simulink model "Week2_Problem3"  (R2020a)
settings: Solver=VariableStepAuto  StartTime=0.0  StopTime=10.0  RelTol=1e-3
settings Model: Creator=sreeram  LastModifiedBy=sreeram

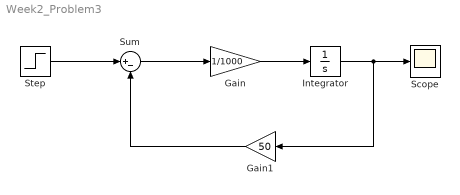
== system Week2_Problem3 ==
  Gain : Gain  Gain=1/1000
  Gain1 : Gain  Gain=50
  Integrator : Integrator
  Scope : Scope
  Step : Step  Time=0  After=500  SampleTime=0
  Sum : Sum  Inputs=|+-
  wires:
  Step/1 -> Sum/1
  Sum/1 -> Gain/1
  Gain/1 -> Integrator/1
  Integrator/1 -> Gain1/1, Scope/1
  Gain1/1 -> Sum/2
